simulink library "intraSpoolingController_ul"  (R2018b)
settings: Solver=VariableStepAuto  StartTime=0.0  StopTime=10.0  RelTol=1e-3
undefined symbols (not defined in the file or in its folder): pathCtrl
settings Model: Creator=James Reed  LastModifiedBy=mcobb

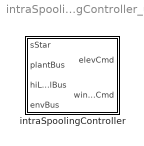
== system intraSpoolingController_ul ==
  intraSpoolingController : Subsystem

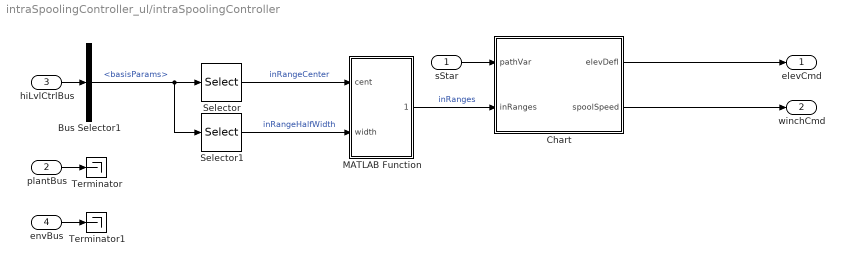
== system intraSpoolingController_ul/intraSpoolingController ==
  "sStar " : Inport
  plantBus : Inport  Port=2  OutDataTypeStr=Bus: plantBus
  hiLvlCtrlBus : Inport  Port=3  OutDataTypeStr=Bus: hiLvlCtrlBus
  envBus : Inport  Port=4  OutDataTypeStr=Bus: envBus
  Bus Selector1 : BusSelector  OutputSignals=basisParams
  Chart : Stateflow chart  TreatAsAtomicUnit=on  mask{outSpoolSpeed=pathCtrl.winchSpeedOut.Value, inSpoolSpeed=pathCtrl.winchSpeedIn.Value, inElevDefl=pathCtrl.elevatorReelInDef.Value}
      mask prompts: outSpoolSpeed "Spool out tether release speed"; inSpoolSpeed "Spool in tether retraction speed"; inElevDefl "Spool in elevator deflection"
  MATLAB Function : MATLAB Function  TreatAsAtomicUnit=on
  Selector : Selector  InputPortWidth=7  IndexOptions=Index vector (dialog)  Indices=6  OutputSizes=1
  Selector1 : Selector  InputPortWidth=7  IndexOptions=Index vector (dialog)  Indices=7  OutputSizes=1
  Terminator : Terminator
  Terminator1 : Terminator
  elevCmd : Outport
  "winchCmd " : Outport  Port=2
  wires:
  Selector1/1 -> MATLAB Function/2(width)  "inRangeHalfWidth"
  MATLAB Function/1(inRanges) -> Chart/2(inRanges)  "inRanges"
  Selector/1 -> MATLAB Function/1(cent)  "inRangeCenter"
  Chart/2(spoolSpeed) -> "winchCmd "/1
  Bus Selector1/1 -> Selector1/1, Selector/1  "<basisParams>"
  hiLvlCtrlBus/1 -> Bus Selector1/1
  Chart/1(elevDefl) -> elevCmd/1
  "sStar "/1 -> Chart/1(pathVar)
  plantBus/1 -> Terminator/1
  envBus/1 -> Terminator1/1

== matlab function intraSpoolingController_ul/intraSpoolingController/MATLAB Function ==
  data: cent input; inRanges output; width input
function inRanges = fcn(cent,width)

inRanges = [...
    cent-width cent+width;...
    0.5+cent-width 0.5+cent+width];

== stateflow chart intraSpoolingController_ul/intraSpoolingController/Chart ==
  state SPOOLOUT
    entry: spoolSpeed = outSpoolSpeed;
    elevDefl = 0;
  state SPOOLIN
    entry: spoolSpeed = inSpoolSpeed;
    elevDefl = inElevDefl;
  (default) -> SPOOLOUT
  SPOOLOUT -> SPOOLIN : [any(and(pathVar>=inRanges(:,1),pathVar<=inRanges(:,2)))]
  SPOOLIN -> SPOOLOUT : [~any(and(pathVar>=inRanges(:,1),pathVar<=inRanges(:,2)))]
  data: pathVar input; inRanges input; inSpoolSpeed parameter; outSpoolSpeed parameter; inElevDefl parameter; elevDefl output; spoolSpeed output
